simulink model "History"  (Simulink 7.4)
settings: Solver=ode45  StartTime=0.0  StopTime=10.0  RelTol=1e-3
settings Model: Creator=dread  LastModifiedBy=dread

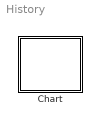
== system History ==
  Chart : Stateflow chart

== stateflow chart Chart ==
  (history)
